simulink model "wipercontrol"  (R2025a)
settings: Solver=VariableStepAuto  StartTime=0.0  StopTime=10.0  RelTol=1e-3
settings Model: DataDictionary=wiperData.sldd  Creator=nikul  LastModifiedBy=nikul

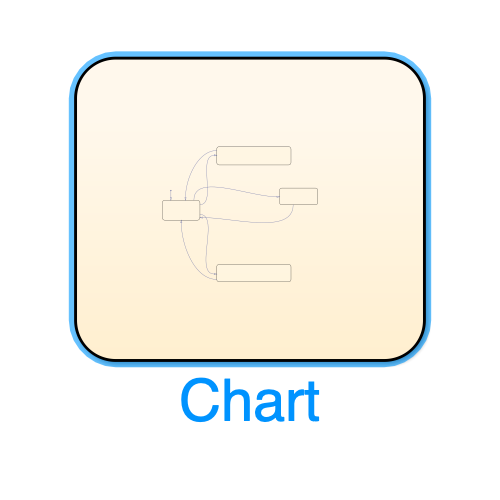
[thumbnail: Simulink's stored preview of the top-level diagram]
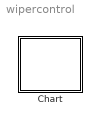
== system wipercontrol ==
  Chart : Stateflow chart  TreatAsAtomicUnit=on

== stateflow chart wipercontrol/Chart ==
  state ?
    state mode_high
      entry:
      Wiper_Speed = WiperSpeed_High;
    state normal
    state Service
    state Mode_intermittent
      state waiting
        entry :
        wiper_speed = 0;
        during:
        timer = timer+1
      state wiping
        entry:
        wiper_speed = wiperspeed_low ;
        timer = 0;
      (default) -> waiting
      waiting -> wiping : [timer >= Intermittent_Delay]
    state Mode_off
      entry:
      Wiper_Speed = 0;
    state mode_low
      entry:
      Wiper_Speed = WiperSpeed_Low;
    normal -> Service : [ServiceMode_Cmd == true]
    mode_high -> Mode_off : [WiperMode_cmd ~= WiperModes.HIGH]
    Mode_off -> mode_high [order 2] : [WiperMode_cmd == WiperModes.High]
    Service -> normal : [ServiceMode_Cmd == false]
    wiping -> waiting : [after(1, sec)]
    Mode_off -> Mode_intermittent [order 1] : [Wipermode_cmd == WiperModes.INTERMITTENT]
    (default) -> Mode_off
    Mode_off -> mode_low [order 3] : [WiperMode_cmd == WiperModes.Low]
    mode_low -> Mode_off : [WiperMode_Cmd ~= WiperModes.LOW]
    Mode_intermittent -> Mode_off : [WiperMode_Cmd ~= WiperModes.INTERMITTENT]
  data: timer local uint8
